simulink model "Overtaking_Integrated"  (R2020b)
settings: Solver=ode23tb  StartTime=0.0  StopTime=25  FixedStep=.01  RelTol=5e-3  EnableMultiTasking=on
InitFcn:
  | %SimulationParameters;
StartFcn:
  | %tic
StopFcn:
  | %toc
  | save(['SimOutputs\' char(datetime('now','Format','y_M_d_HH_mm_ss')) '_' 'sim_out.mat'], 'logsout');
model workspace (MAT data in the model file):
  DLCXref = [-3.2158 4.0142 4.2842 14.7842 29.7842 30.2842 41.7842 46.7842 56.7842]
  DLCYref = [-3.1012 -3.1012 -7.6012 -7.1012 -6.8512 -1.6012 -1.8512 -3.1012 -3.1012]
  Downshift_Speeds = [9.5625 12.9375 16.3125 19.6875 23.0625 26.4375 29.8125 33.1875 36.5625 39.9375 43.3125 46.6875 ... (28 elements, 4x7)]
  EngRevLim = 7000
  Pedal_Positions = [0.1 0.4 0.5 0.9]
  Upshift_Speeds = [12.9375 16.3125 19.6875 33 26.4375 29.8125 33.1875 52.5 39.9375 43.3125 46.6875 77.25 ... (28 elements, 4x7)]
  VEH : object (value not decoded)
values from neighbouring files (symbols this model uses):
  abortTrigger = 0.0    [AOTDataDictionary.sldd]
  Dmax = 3.0    [AOTDataDictionary.sldd]
  dt = 0.05    [AOTDataDictionary.sldd]
  egoVehLength = 4.948    [AOTDataDictionary.sldd]
  egoVehWidth = 2.009    [AOTDataDictionary.sldd]
  gamma = 0.5    [AOTDataDictionary.sldd]
  inflationFactor = 1.1    [AOTDataDictionary.sldd]
  inflexPoint = 0.0    [AOTDataDictionary.sldd]
  L = 3.705    [AOTDataDictionary.sldd]
  npcVehLength = 4.848    [AOTDataDictionary.sldd]
  npcVehWidth = 1.842    [AOTDataDictionary.sldd]
  plotSampleTime = 0.1    [AOTDataDictionary.sldd]
  SenseResolution = 0.1    [AOTDataDictionary.sldd]
  XSenseRange = 20.0    [AOTDataDictionary.sldd]
  YSenseRange = 20.0    [AOTDataDictionary.sldd]
symbols that are objects in the model workspace (value not decoded): VEH
undefined symbols (not defined in the file or in its folder): driving
libraries: simulink x10, drivingscenarioandsensors x5, autolibutils x4, sim3dautolib x3, sim3dlib x2, autolibshared x1, vehdynlibdriver x1, vehdynlibscenariocommon x1, pid_lib x1, vehdynlibsens x1
(part 3 of 3)

== system Overtaking_Integrated/Vehicle Plant/Controllers/Brake Controller/Brake Pressure Control/Bang Bang ABS ==
  Pref : Inport
  Omega : Inport  Port=2
  <Kappa> : Inport  Port=3
  Abs : Abs
  Add : Sum  Inputs=-+
  Bang-bang controller : Subsystem  mask(Sign){}
      mask help: y = sign(x)
      mask Help: Sign Function:\n\t\t\ty = 1 if x > 0\n\t\t\ty = 0 if x = 0\n\t\t\ty = -1 if x < 0
      mask Display: plot(-50,-50,50,50,[-50,50],[0,0],[0,0],[-50,50],[-40,0],[-30,-30],[0,40],[30,30])
  Compare To Constant : simulink/Logic and Bit Operations/Compare To Constant  relop=>=  const=.2  OutDataTypeStr=boolean
  Compare To Constant1 : simulink/Logic and Bit Operations/Compare To Constant  relop=>=  const=.75  OutDataTypeStr=boolean
  Compare To Constant2 : simulink/Logic and Bit Operations/Compare To Constant  relop=>=  const=.5  OutDataTypeStr=boolean
  Constant : Constant  Value=.25
  Debounce : autolibutils/Debounce  DbcOn_Cnts=.1*.001  DbcOff_Cnts=.1*.001  aMode=aMode
      settings: SourceProductBaseCode=PW,MT,UV,VE,VP
  First Order Hold : FirstOrderHold  ErrorTolerance=1
  Gain : Gain  Gain=200
  Logical Operator : Logic  Inputs=3  AllPortsSameDT=off  OutDataTypeStr=boolean
  Rate Transition : RateTransition  Deterministic=off  OutPortSampleTime=.001
  Re/NWheels : Gain  Gain=0.3/4
  Sum of Elements : Sum  Inputs=+
  Switch : Switch  Criteria=u2 > Threshold  ZeroCross=off
  BrkPrsCmd : Outport  VectorParamsAs1DForOutWhenUnconnected=off
  wires:
  Bang-bang controller/1(out_1) -> Gain/1
  Add/1 -> Bang-bang controller/1(in_1)
  First Order Hold/1 -> BrkPrsCmd/1
  <Kappa>/1 -> Rate Transition/1
  Pref/1 -> Switch/3, Compare To Constant1/1  "Pref"
  Constant/1 -> Add/2  "slip ref"
  Switch/1 -> First Order Hold/1
  Rate Transition/1 -> Add/1, Compare To Constant/1
  Logical Operator/1 -> Debounce/1
  Compare To Constant/1 -> Logical Operator/2
  Compare To Constant1/1 -> Logical Operator/3
  Debounce/1 -> Switch/2
  Omega/1 -> Sum of Elements/1
  Abs/1 -> Compare To Constant2/1
  Compare To Constant2/1 -> Logical Operator/1
  Gain/1 -> Switch/1
  Sum of Elements/1 -> Re/NWheels/1
  Re/NWheels/1 -> Abs/1

== system Overtaking_Integrated/Vehicle Plant/Controllers/Brake Controller/Brake Pressure Control/Open Loop ==
  Pref : Inport
  Signal Copy : SignalConversion  OverrideOpt=off
  BrkPrsCmd : Outport  VectorParamsAs1DForOutWhenUnconnected=off
  wires:
  Pref/1 -> Signal Copy/1
  Signal Copy/1 -> BrkPrsCmd/1

== system Overtaking_Integrated/Vehicle Plant/Controllers/ECU/Torque Cmd/Rev Limiter Control ==
  TrqCmd : Inport
  EngSpd : Inport  Port=2
  1-D Lookup Table : Lookup_n-D  NumberOfTableDimensions=1  BreakpointsForDimension1=[1 1.01]  Table=[1 0]  ExtrapMethod=Clip  InternalRulePriority=Speed  RndMeth=Simplest  InputSameDT=on
  Constant : Constant  Value=EngRevLim
  Product : Product
  Product1 : Product  Inputs=*/
  TrqCmdRevLimited : Outport  VectorParamsAs1DForOutWhenUnconnected=off
  wires:
  EngSpd/1 -> Product1/1
  Product/1 -> TrqCmdRevLimited/1
  1-D Lookup Table/1 -> Product/2
  TrqCmd/1 -> Product/1
  Constant/1 -> Product1/2
  Product1/1 -> 1-D Lookup Table/1

== system Overtaking_Integrated/Vehicle Plant/Controllers/Transmission Controller/PRNDL Controller/Shift Controller/calc ==
  note: Determine if next gear will be
      | higher or lower than current gear
  Gear : Inport
  pedal : Inport  Port=2
  VehVel : Inport  Port=3
  f : TriggerPort  TriggerType=function-call  VariantControl=Variant  StatesWhenEnabling=reset
      settings: CopyFcn=Stateflow.SLINSF.SimulinkMan.removeBlockPreDeleteFcn  PreDeleteFcn=Stateflow.SLINSF.SimulinkMan.unsafePredeleteFcn
  Add1 : Sum  Inputs=+-
  Add3 : Sum  Inputs=+-
  Add4 : Sum  Inputs=+-
  Calculate Upshift Threshold : Lookup_n-D  BreakpointsForDimension1=pdlVec  BreakpointsForDimension2=UpGearVec  Table=upShftTbl  ExtrapMethod=Clip  UseLastTableValue=on  InternalRulePriority=Speed  RndMeth=Simplest  InputSameDT=on
      settings: InputPortMap=u0,u1
  Calculate Downshift Threshold : Lookup_n-D  BreakpointsForDimension1=pdlVec  BreakpointsForDimension2=DownGearVec  Table=dwnShftTbl  ExtrapMethod=Clip  UseLastTableValue=on  InternalRulePriority=Speed  RndMeth=Simplest  InputSameDT=on
      settings: InputPortMap=u0,u1
  SpdThr : Outport  VectorParamsAs1DForOutWhenUnconnected=off
  wires:
  pedal/1 -> Calculate Downshift Threshold/1, Calculate Upshift Threshold/1
  Gear/1 -> Calculate Downshift Threshold/2, Calculate Upshift Threshold/2
  Calculate Downshift Threshold/1 -> Add3/2
  Calculate Upshift Threshold/1 -> Add1/1
  VehVel/1 -> Add1/2, Add3/1
  Add1/1 -> Add4/1
  Add3/1 -> Add4/2
  Add4/1 -> SpdThr/1

== system Overtaking_Integrated/Vehicle Plant/Controllers/Transmission Controller/PRNDL Controller/Shift Controller/calc_down ==
  Gear : Inport
  Accel : Inport  Port=2
  f : TriggerPort  TriggerType=function-call  VariantControl=Variant  StatesWhenEnabling=reset
      settings: CopyFcn=Stateflow.SLINSF.SimulinkMan.removeBlockPreDeleteFcn  PreDeleteFcn=Stateflow.SLINSF.SimulinkMan.unsafePredeleteFcn
  Calculate Downshift Threshold : Lookup_n-D  BreakpointsForDimension1=pdlVec  BreakpointsForDimension2=DownGearVec  Table=dwnShftTbl  ExtrapMethod=Clip  UseLastTableValue=on  InternalRulePriority=Speed  RndMeth=Simplest  InputSameDT=on
      settings: InputPortMap=u0,u1
  down_th : Outport  VectorParamsAs1DForOutWhenUnconnected=off
  wires:
  Calculate Downshift Threshold/1 -> down_th/1
  Gear/1 -> Calculate Downshift Threshold/2
  Accel/1 -> Calculate Downshift Threshold/1

== system Overtaking_Integrated/Vehicle Plant/Controllers/Transmission Controller/PRNDL Controller/Shift Controller/calc_up ==
  Gear : Inport
  Accel : Inport  Port=2
  f : TriggerPort  TriggerType=function-call  VariantControl=Variant  StatesWhenEnabling=reset
      settings: CopyFcn=Stateflow.SLINSF.SimulinkMan.removeBlockPreDeleteFcn  PreDeleteFcn=Stateflow.SLINSF.SimulinkMan.unsafePredeleteFcn
  Calculate Upshift Threshold : Lookup_n-D  BreakpointsForDimension1=pdlVec  BreakpointsForDimension2=UpGearVec  Table=upShftTbl  ExtrapMethod=Clip  UseLastTableValue=on  InternalRulePriority=Speed  RndMeth=Simplest  InputSameDT=on
      settings: InputPortMap=u0,u1
  up_th : Outport  VectorParamsAs1DForOutWhenUnconnected=off
  wires:
  Calculate Upshift Threshold/1 -> up_th/1
  Accel/1 -> Calculate Upshift Threshold/1
  Gear/1 -> Calculate Upshift Threshold/2

== system Overtaking_Integrated/Vehicle Plant/Controllers/Transmission Controller/Transmission Controller/TCM ==
  AccCmd : Inport
  EngSpd : Inport  Port=2
  Omega : Inport  Port=3  Unit=rad/s
  function : TriggerPort  TriggerType=function-call  VariantControl=Variant
  Gain : Gain  Gain=.3065/4
  Neutral Select : Subsystem
  Signal Specification1 : SignalSpecification  Unit=m/s
  Signal Specification2 : SignalSpecification  Unit=km/hr
  Speed LPF : DiscreteTransferFcn  Numerator=[0.000000000000000 0.009950166250832 ]  Denominator=[1.000000000000000 -0.990049833749168 ]  mask(DiscretizedDiscreteTransferFcn){}
      mask init:
      | %zoh
  Sum of Elements : Sum  Inputs=+
  TCM Shift Controller : Stateflow chart  TreatAsAtomicUnit=on
  Unit Conversion1 : UnitConversion
  GearCmd : Outport  VectorParamsAs1DForOutWhenUnconnected=off
  wires:
  Signal Specification2/1 -> Speed LPF/1
  TCM Shift Controller/1(GearCmd) -> GearCmd/1  "GearCmd"
  AccCmd/1 -> Neutral Select/1(AccCmd), TCM Shift Controller/2(pedal)  "AccCmd"
  Neutral Select/1(Neutral Select) -> TCM Shift Controller/3(Neutral)
  EngSpd/1 -> Neutral Select/2(EngSpd)
  Speed LPF/1 -> TCM Shift Controller/1(speed)
  Unit Conversion1/1 -> Signal Specification2/1
  Omega/1 -> Sum of Elements/1
  Gain/1 -> Signal Specification1/1
  Signal Specification1/1 -> Unit Conversion1/1
  Sum of Elements/1 -> Gain/1

== system Overtaking_Integrated/Vehicle Plant/Controllers/Brake Controller/Brake Pressure Control/Bang Bang ABS/Bang-bang controller ==
  in_1 : Inport
  Constant : Constant  Value=0
  Data Type Conversion1 : DataTypeConversion  OutDataTypeStr=double  SaturateOnIntegerOverflow=on  RndMeth=Zero
  Data Type Conversion2 : DataTypeConversion  OutDataTypeStr=double  SaturateOnIntegerOverflow=on  RndMeth=Zero
  Relational Operator : RelationalOperator  Operator=>  OutDataTypeStr=boolean  RndMeth=Nearest  InputSameDT=on
  Relational Operator1 : RelationalOperator  Operator=<  OutDataTypeStr=boolean  RndMeth=Nearest  InputSameDT=on
  Sum : Sum  Inputs=+-  InputSameDT=on  SaturateOnIntegerOverflow=on  OutDataTypeStr=Inherit: Same as first input
  out_1 : Outport  InitialOutput=0  VectorParamsAs1DForOutWhenUnconnected=off
  wires:
  Data Type Conversion2/1 -> Sum/2
  Data Type Conversion1/1 -> Sum/1
  Sum/1 -> out_1/1
  Relational Operator/1 -> Data Type Conversion1/1
  Relational Operator1/1 -> Data Type Conversion2/1
  Constant/1 -> Relational Operator/2, Relational Operator1/2
  in_1/1 -> Relational Operator1/1, Relational Operator/1

== system Overtaking_Integrated/Vehicle Plant/Controllers/Transmission Controller/Transmission Controller/TCM/Neutral Select ==
  AccCmd : Inport
  EngSpd : Inport  Port=2
  Constant : Constant  Value=1200
  Constant1 : Constant  Value=1e-2
  Constant2 : Constant  Value=500
  Logical Operator : Logic  AllPortsSameDT=off  OutDataTypeStr=boolean
  Logical Operator1 : Logic  Operator=OR  AllPortsSameDT=off  OutDataTypeStr=boolean
  Relational Operator : RelationalOperator  Operator=<=  OutDataTypeStr=boolean  ZeroCross=off  RndMeth=Simplest
  Relational Operator1 : RelationalOperator  Operator=<=  OutDataTypeStr=boolean  ZeroCross=off  RndMeth=Simplest
  Relational Operator2 : RelationalOperator  Operator=<=  OutDataTypeStr=boolean  ZeroCross=off  RndMeth=Simplest
  Neutral Select : Outport  VectorParamsAs1DForOutWhenUnconnected=off
  wires:
  EngSpd/1 -> Relational Operator/1, Relational Operator2/1
  Relational Operator1/1 -> Logical Operator/1
  AccCmd/1 -> Relational Operator1/1
  Constant1/1 -> Relational Operator1/2
  Logical Operator1/1 -> Neutral Select/1
  Constant/1 -> Relational Operator/2
  Relational Operator/1 -> Logical Operator/2
  Logical Operator/1 -> Logical Operator1/1
  Constant2/1 -> Relational Operator2/2
  Relational Operator2/1 -> Logical Operator1/2

== system Overtaking_Integrated/Vehicle Plant/Controllers/Transmission Controller/Transmission Controller/TCM/TCM Shift Controller/calc ==
  note: Determine if next gear will be
      | higher or lower than current gear
  gear : Inport
  pedal : Inport  Port=2
  speed : Inport  Port=3
  f : TriggerPort  TriggerType=function-call  VariantControl=Variant  StatesWhenEnabling=reset
      settings: CopyFcn=Stateflow.SLINSF.SimulinkMan.removeBlockPreDeleteFcn  PreDeleteFcn=Stateflow.SLINSF.SimulinkMan.unsafePredeleteFcn
  Add1 : Sum  Inputs=+-
  Add3 : Sum  Inputs=+-
  Add4 : Sum  Inputs=+-
  Calculate Upshift Threshold : Lookup_n-D  BreakpointsForDimension1=Pedal_Positions  BreakpointsForDimension2=1:7  Table=Upshift_Speeds  ExtrapMethod=Clip  UseLastTableValue=on  InternalRulePriority=Speed  RndMeth=Simplest  InputSameDT=on
      settings: InputPortMap=u0,u1
  Calculate Downshift Threshold : Lookup_n-D  BreakpointsForDimension1=Pedal_Positions  BreakpointsForDimension2=2:8  Table=Downshift_Speeds  ExtrapMethod=Clip  UseLastTableValue=on  InternalRulePriority=Speed  RndMeth=Simplest  InputSameDT=on
      settings: InputPortMap=u0,u1
  SpdThr : Outport  VectorParamsAs1DForOutWhenUnconnected=off
  wires:
  pedal/1 -> Calculate Downshift Threshold/1, Calculate Upshift Threshold/1
  gear/1 -> Calculate Downshift Threshold/2, Calculate Upshift Threshold/2
  Calculate Downshift Threshold/1 -> Add3/2
  Calculate Upshift Threshold/1 -> Add1/1
  speed/1 -> Add1/2, Add3/1
  Add1/1 -> Add4/1
  Add3/1 -> Add4/2
  Add4/1 -> SpdThr/1

== system Overtaking_Integrated/Vehicle Plant/Controllers/Transmission Controller/Transmission Controller/TCM/TCM Shift Controller/calc_down ==
  gear : Inport
  pedal : Inport  Port=2
  f : TriggerPort  TriggerType=function-call  VariantControl=Variant  StatesWhenEnabling=reset
      settings: CopyFcn=Stateflow.SLINSF.SimulinkMan.removeBlockPreDeleteFcn  PreDeleteFcn=Stateflow.SLINSF.SimulinkMan.unsafePredeleteFcn
  Calculate Downshift Threshold : Lookup_n-D  BreakpointsForDimension1=Pedal_Positions  BreakpointsForDimension2=2:8  Table=Downshift_Speeds  ExtrapMethod=Clip  UseLastTableValue=on  InternalRulePriority=Speed  RndMeth=Simplest  InputSameDT=on
      settings: InputPortMap=u0,u1
  down_th : Outport  VectorParamsAs1DForOutWhenUnconnected=off
  wires:
  Calculate Downshift Threshold/1 -> down_th/1
  gear/1 -> Calculate Downshift Threshold/2
  pedal/1 -> Calculate Downshift Threshold/1

== system Overtaking_Integrated/Vehicle Plant/Controllers/Transmission Controller/Transmission Controller/TCM/TCM Shift Controller/calc_up ==
  gear : Inport
  pedal : Inport  Port=2
  f : TriggerPort  TriggerType=function-call  VariantControl=Variant  StatesWhenEnabling=reset
      settings: CopyFcn=Stateflow.SLINSF.SimulinkMan.removeBlockPreDeleteFcn  PreDeleteFcn=Stateflow.SLINSF.SimulinkMan.unsafePredeleteFcn
  Calculate Upshift Threshold : Lookup_n-D  BreakpointsForDimension1=Pedal_Positions  BreakpointsForDimension2=1:7  Table=Upshift_Speeds  ExtrapMethod=Clip  UseLastTableValue=on  InternalRulePriority=Speed  RndMeth=Simplest  InputSameDT=on
      settings: InputPortMap=u0,u1
  up_th : Outport  VectorParamsAs1DForOutWhenUnconnected=off
  wires:
  Calculate Upshift Threshold/1 -> up_th/1
  pedal/1 -> Calculate Upshift Threshold/1
  gear/1 -> Calculate Upshift Threshold/2

== stateflow chart Overtaking_Integrated/Vehicle Plant/Controllers/Transmission Controller/Transmission Controller/TCM/TCM Shift Controller ==
  settings: sampleTime=0.01
  state GearCmd [parallel]
    settings: executionOrder=1
    state Neutral
      en:
      GearCmd = 0;
    state G1
      en:
      GearCmd = 1;
    state G2
      en:
      GearCmd = 2;
      du:
      [SpdThr] = calc(2,pedal,speed);
    state G3
      en:
      GearCmd = 3;
      du:
      [SpdThr] = calc(3,pedal,speed);
    state G8
      en:
      GearCmd = 8;
    state G7
      en:
      GearCmd = 7;
    state G6
      en:
      GearCmd = 6;
    state G5
      en:GearCmd=5;
      du:[SpdThr]=calc(5,pedal,speed);
    state G4
      en:
      GearCmd = 4;
      du:
      [SpdThr] = calc(4,pedal,speed);
    (default) -> Neutral
    Neutral -> G1 : [~Neutral]
    G1 -> G2 [order 1] : Up
    G2 -> G3 [order 1] : Up
    G1 -> Neutral [order 2] : [Neutral]
    G2 -> G1 [order 2] : Down
    G3 -> G2 [order 2] : Down
    G3 -> G4 [order 1] : Up
    G4 -> G3 [order 2] : Down
    G7 -> G8 [order 1] : Up
    G5 -> G6 [order 1] : Up
    G6 -> G7 [order 1] : Up
    G4 -> G5 [order 1] : Up
    G5 -> G4 [order 2] : Down
    G6 -> G5 [order 2] : Down
    G7 -> G6 [order 2] : Down
    G8 -> G7 : Down
  state SelectionState [parallel]
    du:[up_th]=calc_up(GearCmd,pedal);
    du:[down_th]=calc_down(GearCmd,pedal);
    settings: executionOrder=2
    state SteadyState
      en:
      clutchControl = 0;
    state preDownShifting
    state preUpShifting
    state UpShifting
      en:
      GearCmd = GearCmd + 0.5;
    state DownShifting
      en:
      GearCmd = GearCmd - 0.5;
    (default) -> SteadyState
    SteadyState -> (junction 62) [order 1] : [speed < down_th && ...
        | GearCmd >1]
    SteadyState -> (junction 128) [order 2] : [speed > up_th &&...
        | GearCmd <= 5 && ...
        | floor(GearCmd) == GearCmd]
    (junction 62) -> preDownShifting
    (junction 128) -> preUpShifting
    (junction 168) -> SteadyState
    (junction 23) -> SteadyState
    (junction 161) -> SteadyState
    preDownShifting -> (junction 168) [order 2] : [speed >= down_th]
    preUpShifting -> (junction 161) [order 2] : [speed <= up_th]
    preUpShifting -> UpShifting [order 1] : after(0.5,sec)
        | [speed>up_th]
    preDownShifting -> DownShifting [order 1] : after(0.5, sec)
        | [speed < down_th - 2]
    DownShifting -> (junction 23) : {GearCmd.Down;}
    UpShifting -> (junction 23) : {GearCmd.Up;}
  state up_th = calc_up(gear,pedal) [function]
  state down_th = calc_down(gear,pedal) [function]
  state SpdThr = calc(gear,pedal,speed) [function]
  data: gear function_input; pedal function_input; up_th function_output; gear function_input; pedal function_input; down_th function_output; gear function_input; pedal function_input; SpdThr function_output; speed function_input; GearCmd output int8; speed input; pedal input; clutchControl local double; SpdThr local double; Neutral input; up_th local double; down_th local double
  events: Up local EITHER_EDGE_EVENT; Down local EITHER_EDGE_EVENT

== matlab function Overtaking_Integrated/Plotting/MATLAB Function ==
  data: npcVehPgonsWorld output Bus: VehPgons; npcVehPgonsEgo input; VehFdbk_ISO input
function npcVehPgonsWorld = fcn(npcVehPgonsEgo, VehFdbk_ISO)

npcVehPgonsWorld.NumVeh = npcVehPgonsEgo.NumVeh; 

for i = 1:npcVehPgonsEgo.NumVeh
    for j = 1:length(npcVehPgonsEgo.VehPgon(i,1).X)
        inputPose.X = npcVehPgonsEgo.VehPgon(i,1).X(j,1);inputPose.Y = npcVehPgonsEgo.VehPgon(i,1).Y(j,1);inputPose.Z = 0;
        outputPose = transformEgo(inputPose, VehFdbk_ISO.Position, VehFdbk_ISO.Orientation, 1);
        npcVehPgonsWorld.VehPgon(i,1).X(j,1) = outputPose.X;
        npcVehPgonsWorld.VehPgon(i,1).Y(j,1) = outputPose.Y;
    end
    
end

== matlab function Overtaking_Integrated/ScenarioSetup/GenerateNPCPolygons/GenerateObstaclepolygons1 ==
  data: ActorsEgo input; npcVehPgons output Bus: VehPgons; npcVehLength parameter; npcVehWidth parameter; egoVehLength parameter; egoVehWidth parameter; VehFdbk_ISO input; npcVehPgonsWorld output Bus: VehPgons
function [npcVehPgons, npcVehPgonsWorld] = fcn(ActorsEgo, npcVehLength, npcVehWidth, egoVehLength, egoVehWidth, VehFdbk_ISO)
coder.extrinsic('generateObstclPgon');
[npcVehPgons, npcVehPgonsWorld] = generateObstclPgon(ActorsEgo, npcVehLength, npcVehWidth, egoVehLength, egoVehWidth, VehFdbk_ISO);

== stateflow chart Overtaking_Integrated/Vehicle Plant/Controllers/Transmission Controller/PRNDL Controller/Shift Controller ==
  settings: sampleTime=0.01
  state GearSelect [parallel]
    settings: executionOrder=1
    state Reverse
      entry:
      GearState = -1;
    state Neutral
      entry:
      GearState = 0;
    state Odd
      en:GearState = Gear;
      du:[SpdThr]=calc(Gear,Accel,VehVel);
    state Even
      en:GearState = Gear;
      du:[SpdThr]=calc(Gear,Accel,VehVel);
    state Park
      entry:
      GearState = 80;
    (default) -> (junction 461) : /* InitialGear */
        | {Gear = GearInit;}
    (junction 461) -> (junction 463) [order 1] : [GearInit==80]
    (junction 463) -> Park
    (junction 461) -> (junction 441) [order 2]
    (junction 441) -> (junction 442) [order 1] : [GearInit<0]
    (junction 442) -> Reverse
    (junction 441) -> (junction 457) [order 2]
    (junction 457) -> (junction 459) [order 1] : [GearInit==0]
    (junction 459) -> Neutral
    (junction 457) -> (junction 445) [order 2]
    (junction 445) -> (junction 446) [order 1] : [GearInit%%2==0]
    (junction 445) -> Odd [order 2]
    (junction 446) -> Even
    (junction 363) -> (junction 366)
    (junction 366) -> Odd
    Even -> (junction 363) [order 1] : UP
        | {Gear=Gear+1;}
    Neutral -> Reverse [order 2] : [PRNDL==-1]
        | {Gear=-1;}
    Neutral -> Odd [order 1] : UP
        | {Gear=Gear+1;}
    Odd -> Even [order 1] : UP
        | {Gear=Gear+1;}
    Reverse -> Neutral : [PRNDL==1]
        | {Gear=1;}
    Even -> Odd [order 2] : DOWN
        | {Gear=Gear-1;}
    Neutral -> (junction 380) [order 3]
    (junction 379) -> Neutral
    (junction 370) -> Neutral
    Odd -> (junction 361) [order 2] : DOWN
        | {Gear=Gear-1;}
    (junction 357) -> Even
    Even -> (junction 371) [order 3] : [Gear==0]
    (junction 361) -> (junction 357)
    (junction 380) -> Park : after(tPark,sec)
        | [PRNDL==80 &&...
        | Brake>0.5&&...
        | abs(VehVel)<=1&&...
        | Accel<=0.05]
    Park -> (junction 379) : [abs(VehVel)<=1&&Accel>0]
    (junction 371) -> (junction 370)
  state SelectionState [parallel]
    du:[up_th]=calc_up(GearState,Accel);
    du:[down_th]=calc_down(GearState,Accel);
    settings: executionOrder=2
    state Inactive
    state SteadyState
      en:
      clutchControl = 0;
    state preUpShifting
      en:clutchControl = 1;
    state preDownShifting
      en:clutchControl = 1;
    state UpShifting
      en:
      GearState = GearState + 0.5;
    state DownShifting
      en:
      GearState = GearState - 0.5;
    (default) -> (junction 514)
    (junction 514) -> Inactive [order 2]
    (junction 514) -> SteadyState [order 1] : [PRNDL==1]
    (junction 517) -> Inactive
    Inactive -> (junction 520) : [PRNDL==1]
    SteadyState -> (junction 517) [order 3] : [PRNDL~=1]
    SteadyState -> (junction 62) [order 2] : [GearState >0&&...
        | (VehVel < down_th ||...
        |  EngSpd<1200)]
    (junction 62) -> preDownShifting
    (junction 520) -> SteadyState
    SteadyState -> (junction 128) [order 1] : [Accel>0 && (abs(VehVel) > up_th) &&...
        | (GearState <= N ) &&...
        | (floor(GearState) == GearState) &&...
        | (EngSpd>=2000)]
    (junction 128) -> preUpShifting
    (junction 168) -> SteadyState
    (junction 23) -> SteadyState
    (junction 161) -> SteadyState
    preDownShifting -> (junction 168) [order 2] : [VehVel >= down_th &&...
        | EngSpd>2000]
    preUpShifting -> (junction 161) [order 2] : [VehVel <= up_th ||...
        |  EngSpd<1200]
    preUpShifting -> UpShifting [order 1] : after(tClutch,sec)
        | [VehVel>up_th]
    preDownShifting -> DownShifting [order 1] : after(tClutch, sec)
        | [(VehVel < down_th - 2) || VehVel<=0 ||EngSpd<750]
    DownShifting -> (junction 23) : {GearSelect.DOWN;}
    UpShifting -> (junction 23) : {GearSelect.UP;}
  state up_th = calc_up(Gear,Accel) [function]
  state down_th = calc_down(Gear,Accel) [function]
  state SpdThr = calc(Gear,pedal,VehVel) [function]
  data: Gear function_input; Accel function_input; up_th function_output; Gear function_input; Accel function_input; down_th function_output; Gear function_input; pedal function_input; SpdThr function_output; VehVel function_input; PRNDL input; Gear output double =GearInit; clutchControl output double; Accel input; Brake input; EngSpd input; VehVel input; SpdThr local double; up_th local double; down_th local double; tPark parameter; tRev parameter; GearInit parameter double; N local double =size(upShftTbl,2); tClutch parameter; GearState local double
  events: DOWN local EITHER_EDGE_EVENT; UP local EITHER_EDGE_EVENT

== matlab function Overtaking_Integrated/ScenarioSetup/Scenario Reader/Pack Ego Actor ==
  data: pos input; egoActor output Bus: BusActorsActors size=1; vel input; yaw input; yawRate input
function egoActor = packEgo(pos,vel,yaw,yawRate)
% Pack ego information into a single ego actor bus
%
% Imoprtant note:
% Output is a bus of type BusActorsActors. This is the same bus used by the
% Scenario Reader to output an individual actor. If you change the
% output bus name of Scenario Reader, change the output bus name here
% as well by clicking on 'Edit Data' in the menu above.

egoActor = struct(...
    'ActorID',2,...
    'Position', [pos(1) pos(2) 0], ...
    'Velocity', [vel(1) vel(2) 0], ...
    'Roll', 0, ...
    'Pitch', 0, ...
    'Yaw', yaw, ...
    'AngularVelocity', [0 0 yawRate]);

== matlab function Overtaking_Integrated/Plotting/Plot ==
  data: XSenseRange parameter; YSenseRange parameter; SenseResolution parameter; egoVehLength parameter; egoVehWidth parameter; VehFdbk_ISO input; ActorsEgo input; Lanes input; npcVehPgons input; safeSetEgo input; safeRiskMapEgo input; reachableSetEgo input; SRSetEgo input; XPredictedWorld input; XmpcRefWorld input; MVPredictedWorld input; ReferenceGoal input; MpcOAConstraints input; npcVehPgonsWorld input
function fcn(XSenseRange, YSenseRange, SenseResolution, egoVehLength, egoVehWidth, VehFdbk_ISO, ActorsEgo, Lanes, npcVehPgons, safeSetEgo, safeRiskMapEgo, reachableSetEgo, SRSetEgo, XPredictedWorld, XmpcRefWorld, MVPredictedWorld, ReferenceGoal, MpcOAConstraints, npcVehPgonsWorld)

coder.extrinsic('plot_all');

plot_all(XSenseRange, YSenseRange, SenseResolution,egoVehLength, egoVehWidth, VehFdbk_ISO, ActorsEgo, Lanes, npcVehPgons, safeSetEgo, safeRiskMapEgo, reachableSetEgo, SRSetEgo, XPredictedWorld,XmpcRefWorld, MVPredictedWorld, ReferenceGoal,MpcOAConstraints);

== matlab function Overtaking_Integrated/ScenarioSetup/GenerateNPCPolygons/GenerateObstaclepolygons ==
  data: ActorsEgo input; VehFdbk_ISO input; npcVehPgons output Bus: VehPgons; npcVehLength parameter; npcVehWidth parameter; egoVehLength parameter; egoVehWidth parameter; Dmax parameter; gamma parameter; inflexPoint parameter; inflationFactor parameter
function npcVehPgons = fcn(ActorsEgo,VehFdbk_ISO,...
                            npcVehLength, npcVehWidth, egoVehLength, egoVehWidth, Dmax, gamma, inflexPoint,inflationFactor)
coder.extrinsic('generateObstclPgon');
npcVehPgons = generateObstclPgon(npcVehLength, npcVehWidth, egoVehLength, egoVehWidth, Dmax, gamma, inflexPoint,inflationFactor,...
                                            ActorsEgo,VehFdbk_ISO);
